simulink model "stellaris_test_gpio"  (R2012b)
settings: Solver=FixedStepDiscrete  SolverMode=SingleTasking  StartTime=0.0  StopTime=10.0  FixedStep=0.001  RelTol=1e-3
libraries: stellaris_lib x9, simulink x3
settings Model: Creator=peselnikmg  LastModifiedBy=peselnikmg
settings DataIOCC: SignalLoggingSaveFormat=ModelDataLogs
settings OptimizationCC: OptimizeModelRefInitCode=on  LifeSpan=1
settings HardwareCC: ProdEndianess=LittleEndian  ProdHWDeviceType=Texas Instruments->TMS470
settings RTWCC: SystemTargetFile=stellaris.tlc  TemplateMakefile=stellaris_tmf  PostCodeGenCommand=stellaris_customcode(buildInfo)  Description=TI Stellaris LaunchPad  GenerateReport=on  ProcessScript=stellaris_make_rtw_hook  IncludeHyperlinkInReport=on  GenerateTraceInfo=on  GenerateTraceReport=on  GenerateTraceReportSl=on  GenerateTraceReportSf=on  GenerateTraceReportEml=on  GenerateCodeMetricsReport=on  GenerateCodeReplacementReport=on
settings CodeAppCC: IgnoreCustomStorageClasses=off
settings STFCustomTargetCC: CodeReplacementLibrary=ANSI_C  CombineOutputUpdateFcns=on  ERTCustomFileBanners=on  SupportContinuousTime=off  SupportNonInlinedSFcns=off  GRTInterface=off  SystemTargetFile=stellaris.tlc
settings ERTTargetCC: CodeReplacementLibrary=ANSI_C  MultiwordLength=2048  ParMdlRefBuildCompliant=off  CompOptLevelCompliant=off  ConcurrentExecutionCompliant=off  ERTFirstTimeCompliant=off  ModelStepFunctionPrototypeControlCompliant=off  CPPClassGenCompliant=off  InlinedParameterPlacement=NonHierarchical  ERTCustomFileTemplate=stellaris_srmain.tlc  ConvertIfToSwitch=off  SuppressUnreachableDefaultCases=off

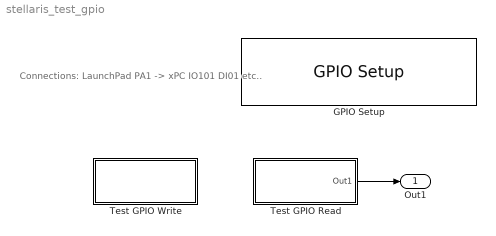
== system stellaris_test_gpio ==
  note: Connections:
      | LaunchPad PA1 -> xPC IO101 DI01
      | etc..
  GPIO Setup : stellaris_lib/GPIO/GPIO Setup  GPIO_PORTX_BASE=GPIO_PORTA_BASE  PinsOutput_0=Input  PinsOutput_1=Input  PinsOutput_2=Output  PinsOutput_3=Output  PinsOutput_4=Output  PinsOutput_5=Input  PinsOutput_6=Input  PinsOutput_7=Input
  Test GPIO Read : Subsystem  Priority=2  TreatAsAtomicUnit=on
      settings: AttributesFormatString=Priority: %<Priority>
  Test GPIO Write : Subsystem  Priority=1  TreatAsAtomicUnit=on
      settings: AttributesFormatString=Priority: %<Priority>
  Out1 : Outport
  wires:
  Test GPIO Read/1(Out1) -> Out1/1

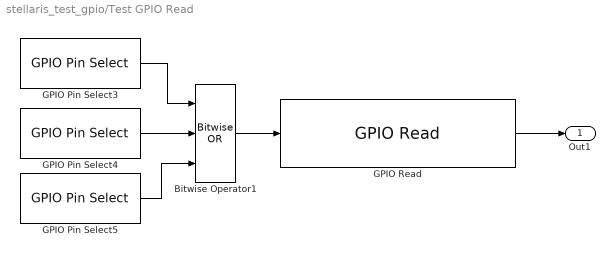
== system stellaris_test_gpio/Test GPIO Read ==
  Bitwise Operator1 : simulink/Logic and Bit Operations/Bitwise Operator  logicop=OR  UseBitMask=off  NumInputPorts=3  BitMask=bin2dec('11011001')  BitMaskRealWorld=Stored Integer
  GPIO Pin Select3 : stellaris_lib/GPIO/GPIO Pin Select  GPIO_PIN_X=GPIO_PIN_2
  GPIO Pin Select4 : stellaris_lib/GPIO/GPIO Pin Select  GPIO_PIN_X=GPIO_PIN_3
  GPIO Pin Select5 : stellaris_lib/GPIO/GPIO Pin Select  GPIO_PIN_X=GPIO_PIN_4
  GPIO Read : stellaris_lib/GPIO/GPIO Read  GPIO_PORTX_BASE=GPIO_PORTA_BASE
  Out1 : Outport
  wires:
  GPIO Pin Select4/1 -> Bitwise Operator1/2
  GPIO Pin Select3/1 -> Bitwise Operator1/1
  GPIO Pin Select5/1 -> Bitwise Operator1/3
  Bitwise Operator1/1 -> GPIO Read/1
  GPIO Read/1 -> Out1/1

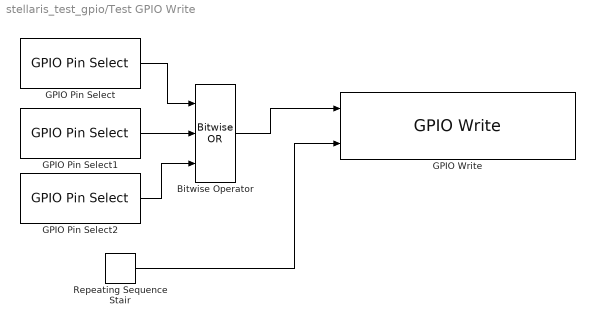
== system stellaris_test_gpio/Test GPIO Write ==
  Bitwise Operator : simulink/Logic and Bit Operations/Bitwise Operator  logicop=OR  UseBitMask=off  NumInputPorts=3  BitMask=bin2dec('11011001')  BitMaskRealWorld=Stored Integer
  GPIO Pin Select : stellaris_lib/GPIO/GPIO Pin Select  GPIO_PIN_X=GPIO_PIN_2
  GPIO Pin Select1 : stellaris_lib/GPIO/GPIO Pin Select  GPIO_PIN_X=GPIO_PIN_3
  GPIO Pin Select2 : stellaris_lib/GPIO/GPIO Pin Select  GPIO_PIN_X=GPIO_PIN_4
  GPIO Write : stellaris_lib/GPIO/GPIO Write  GPIO_PORTX_BASE=GPIO_PORTA_BASE
  Repeating Sequence Stair : simulink/Sources/Repeating Sequence Stair  OutValues=[0 4 8 16].'  tsamp=0.05  OutMin=[]  OutMax=[]  OutDataTypeStr=uint8  OutputDataTypeScalingMode=uint8  OutDataType=fixdt(0,8)  ConRadixGroup=Best Precision: Vector-wise  OutScaling=2^-12
  wires:
  Bitwise Operator/1 -> GPIO Write/1
  GPIO Pin Select1/1 -> Bitwise Operator/2
  GPIO Pin Select/1 -> Bitwise Operator/1
  Repeating Sequence Stair/1 -> GPIO Write/2
  GPIO Pin Select2/1 -> Bitwise Operator/3
